simulink model "Model3_raspLin"  (R2023a)
settings: Solver=VariableStepAuto  StartTime=0.0  StopTime=100  RelTol=1e-3
undefined symbols (not defined in the file or in its folder): A_lin, B_lin, C_lin, D_lin, param, ustarr, xstarr, ystarr
settings Model: Creator=Admin  LastModifiedBy=Admin

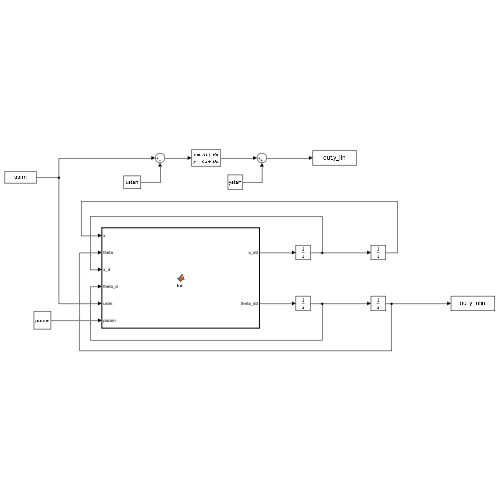
[thumbnail: Simulink's stored preview of the top-level diagram]
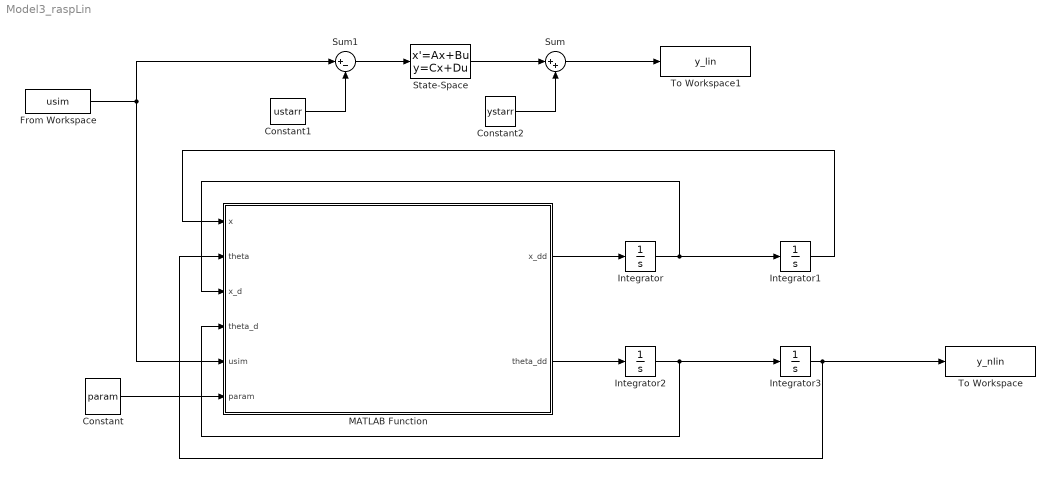
== system Model3_raspLin ==
  Constant : Constant  Value=param  OutDataTypeStr=Bus: par_bus
  Constant1 : Constant  Value=ustarr
  Constant2 : Constant  Value=ystarr
  From Workspace : FromWorkspace  VariableName=usim
  Integrator{,1..3} (4 alike) : Integrator
  MATLAB Function : MATLAB Function  TreatAsAtomicUnit=on
  State-Space : StateSpace  A=A_lin  B=B_lin  C=C_lin  D=D_lin  InitialCondition=-xstarr
  Sum : Sum  Inputs=|++
  Sum1 : Sum  Inputs=|+-
  To Workspace : ToWorkspace  VariableName=y_nlin  SaveFormat=Timeseries  SampleTime=-1
      settings: Save2DSignal=2-D array (concatenate along first dimension)
  To Workspace1 : ToWorkspace  VariableName=y_lin  SaveFormat=Timeseries  SampleTime=-1
      settings: Save2DSignal=2-D array (concatenate along first dimension)
  wires:
  Constant/1 -> MATLAB Function/6(param)
  MATLAB Function/1(x_dd) -> Integrator/1
  MATLAB Function/2(theta_dd) -> Integrator2/1
  Integrator/1 -> Integrator1/1, MATLAB Function/3(x_d)
  Integrator1/1 -> MATLAB Function/1(x)
  Integrator2/1 -> Integrator3/1, MATLAB Function/4(theta_d)
  Integrator3/1 -> To Workspace/1, MATLAB Function/2(theta)
  From Workspace/1 -> Sum1/1, MATLAB Function/5(usim)
  Constant1/1 -> Sum1/2
  Constant2/1 -> Sum/2
  Sum1/1 -> State-Space/1
  State-Space/1 -> Sum/1
  Sum/1 -> To Workspace1/1

== matlab function Model3_raspLin/MATLAB Function ==
  data: x input; x_dd output; theta input; x_d input; theta_d input; usim input; param input; theta_dd output
function [x_dd, theta_dd] = fcn(x, theta, x_d, theta_d, usim, param)
x_dd = (param.l0 + x)*theta_d^2 - (param.k/param.m)*x + param.g*cos(theta) - param.csi*x_d;
theta_dd = (-param.g/(param.l0 + x))*sin(theta) - ((2*x_d)/(param.l0 + x))*theta_d - param.csi*theta_d + usim/(param.m*((param.l0+x)^2)); 
end
